simulink model "simulinkkkk"  (R2022a)
settings: Solver=VariableStepAuto  StartTime=0.0  StopTime=3  RelTol=1e-3
values from neighbouring files (symbols this model uses):
  Cd = c2d(C,Tc,'tustin')    [es20210205.m]
  den = conv(den1,den2)    [es20210205.m]
  num = [10 1]*1000    [es20210205.m]
  Tc = 0.001    [es20210205.m]
settings Model: Creator=Stefano  LastModifiedBy=Stefano

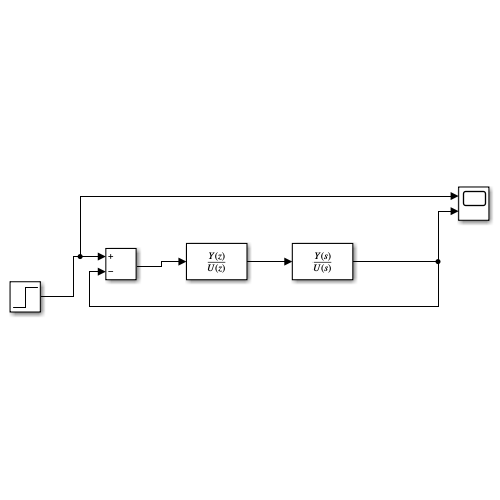
[thumbnail: Simulink's stored preview of the top-level diagram]
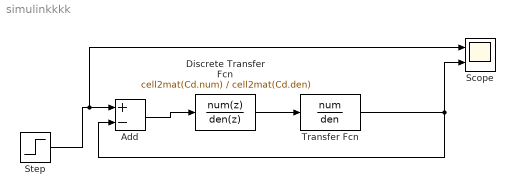
== system simulinkkkk ==
  Add : Sum  Inputs=+-
  Discrete Transfer Fcn : DiscreteTransferFcn  Numerator=cell2mat(Cd.num)  Denominator=cell2mat(Cd.den)  SampleTime=Tc
  Scope : Scope  NumInputPorts=2
  Step : Step  SampleTime=0
  Transfer Fcn : TransferFcn  Numerator=num  Denominator=den
  wires:
  Discrete Transfer Fcn/1 -> Transfer Fcn/1
  Transfer Fcn/1 -> Add/2, Scope/2
  Step/1 -> Scope/1, Add/1
  Add/1 -> Discrete Transfer Fcn/1
